simulink model "ReverbEffect"  (R2020a)
settings: Solver=VariableStepAuto  StartTime=0.0  StopTime=10.0  RelTol=1e-3
libraries: simulink x2, dspsnks4 x1, dspvision x1
settings Model: Creator=Administrator  LastModifiedBy=Administrator

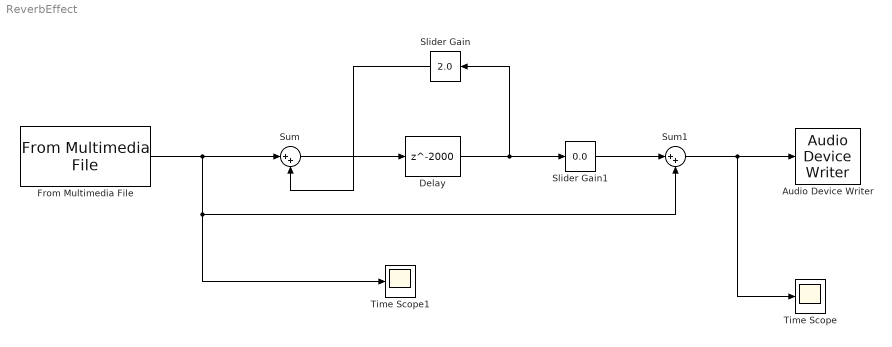
== system ReverbEffect ==
  Audio Device Writer : dspsnks4/Audio Device Writer  Driver=DirectSound  Device=Default  InheritSampleRate=on  SampleRate=44100  BitDepth=16-bit integer  BufferSize=4096  NumBuffers=10  DefaultOutputChannelMapping=on  OutputChannelMapping=1:2  OutputNumUnderrunSamples=off  DriverIdx=1  DeviceWarnFlag=''
  Delay : Delay  DelayLength=2000  InitialCondition=0  UseCircularBuffer=on
  From Multimedia File : dspvision/From Multimedia File  inputFilename=C:\Program Files\Polyspace\toolbox\dsp\dsp\audio48kHz.wav  readRange=[1 Inf]  loop=on  numPlays=inf  outputStreams=Audio only  videoDataType=single  audioDataType=double  inheritSampleTime=on  userDefinedSampleTime=1/30  noAudioOutput=off  isIntensityVideo=off  fourcc=RGB  colorVideoFormat=Separate color signals  outputEOF=off  dataOrg=Column-major  audioFrameSize=1024  computeAudioFrameSize=off  outSamplingMode=Sample based
  Slider Gain : simulink/Math Operations/Slider Gain  gain=2.0  low=0  high=2
  Slider Gain1 : simulink/Math Operations/Slider Gain  gain=0.0  low=0  high=2
  Sum : Sum  Inputs=|++
  Sum1 : Sum  Inputs=|++
  Time Scope : Scope
  Time Scope1 : Scope
  wires:
  Delay/1 -> Slider Gain/1, Slider Gain1/1
  Slider Gain1/1 -> Sum1/1
  From Multimedia File/1 -> Time Scope1/1, Sum1/2, Sum/1
  Sum/1 -> Delay/1
  Slider Gain/1 -> Sum/2
  Sum1/1 -> Time Scope/1, Audio Device Writer/1
